simulink model "active_cell_balancing"  (R2021a)
settings: Solver=VariableStepAuto  StartTime=0.0  StopTime=5  RelTol=1e-3
undefined symbols (not defined in the file): Ion, Lithium
libraries: spsIdealSwitchLib x4, spsSeriesRLCBranchLib x4, spsBatteryLib x2, spsDiodeLib x2, spsDCVoltageSourceLib x1, spsGroundLib x1, spsPWMGenerator2LevelLib x1, spspowerguiLib x1
settings Model: Creator=suraj kumar  LastModifiedBy=suraj kumar

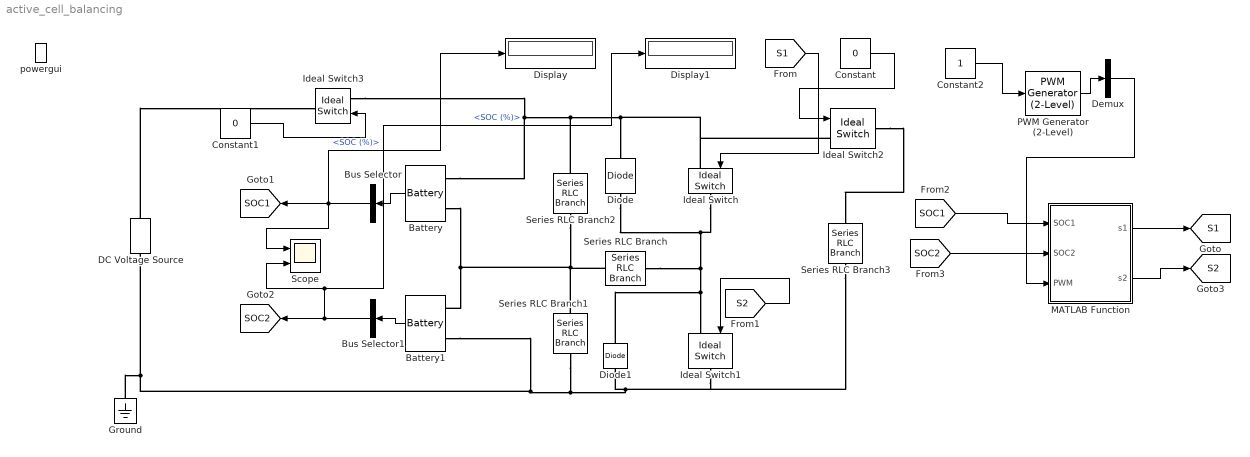
== system active_cell_balancing ==
  Battery : spsBatteryLib/Battery  BatType=Lithium-Ion  ShowTempParam=off  ThermalPreset=no  ShowAgeParam=off  NomV=3.6  NomQ=5.4  SOC=50  Batt_Tr=30  PresetModel=on  MaxQ=5.4  MinV=2.7  FullV=4.1904  Dis_rate=2.3478  R=0.0066667  Normal_OP=4.8835  expZone="[3.8894      0.2653]"  current=[6.5 13 32.5]  Units=Time  Tci=20  NomT=20  T2=-30  MaxQ2=4.8  FullV2=7.1  Normal_OP2=5.655  expZone2="[6.58           1]"  Rca=0.6  ti=2000  Dp=0  Neq0=0  Tsim=1e6  Ta1=25  Qeol=5.4*0.9  Reol=0.013333*1.2  Char_age=[2.3478, 3]  Dis_age=[2.3478, 10]  N1=1500  N2=10500  N3=1000  N4=1400  Ta2=45  N5=950
  Battery1 : spsBatteryLib/Battery  BatType=Lithium-Ion  ShowTempParam=off  ThermalPreset=no  ShowAgeParam=off  NomV=3.7  NomQ=5.4  SOC=60  Batt_Tr=30  PresetModel=on  MaxQ=5.4  MinV=2.775  FullV=4.3068  Dis_rate=2.3478  R=0.0068519  Normal_OP=4.8835  expZone="[3.9974      0.2653]"  current=[6.5 13 32.5]  Units=Time  Tci=20  NomT=20  T2=-30  MaxQ2=4.8  FullV2=7.1  Normal_OP2=5.655  expZone2="[6.58           1]"  Rca=0.6  ti=2000  Dp=0  Neq0=0  Tsim=1e6  Ta1=25  Qeol=5.4*0.9  Reol=0.013333*1.2  Char_age=[2.3478, 3]  Dis_age=[2.3478, 10]  N1=1500  N2=10500  N3=1000  N4=1400  Ta2=45  N5=950
  Bus Selector : BusSelector  OutputSignals=SOC (%)
  Bus Selector1 : BusSelector  OutputSignals=SOC (%)
  Constant : Constant  Value=0
  Constant1 : Constant  Value=0
  Constant2 : Constant
  DC Voltage Source : spsDCVoltageSourceLib/DC Voltage Source  Amplitude=12  Measurements=None
  Demux : Demux  Outputs=1
  Diode : spsDiodeLib/Diode  Ron=0.001  Lon=0  Vf=0.8  IC=0  UseSnubber=0  Rs=500  Cs=250e-9  Measurements=off
  Diode1 : spsDiodeLib/Diode  Ron=0.001  Lon=0  Vf=0.8  IC=0  UseSnubber=0  Rs=500  Cs=250e-9  Measurements=off
  Display : Display
  Display1 : Display
  Ground : spsGroundLib/Ground  LConnTagsString=a
  Ideal Switch{,1..3} (4 alike) : spsIdealSwitchLib/Ideal Switch  Ron=0.001  Lon=0  IC=0  Rs=1e5  Cs=inf  Measurements=off
  MATLAB Function : MATLAB Function  TreatAsAtomicUnit=on
  PWM Generator (2-Level) : spsPWMGenerator2LevelLib/PWM Generator (2-Level)  ModulatorType=Single-phase half-bridge (2 pulses)  ModulatorMode=Unsynchronized  Fc=500  Pc=0  nF=27  MinMax="[ -1  1 ]"  SamplingTechnique=Natural  ModulatingSignals=off  m=0.8  Freq=60  Phase=0  Ts=0  ShowCarrierOutport=off
  Scope : Scope  NumInputPorts=2
  Series RLC Branch : spsSeriesRLCBranchLib/Series RLC Branch  LConnTagsString=__new0  RConnTagsString=__new0  BranchType=L  Resistance=1  Inductance=1e-3  SetiL0=off  InitialCurrent=0  Capacitance=1e-6  Setx0=off  InitialVoltage=0  Measurements=None
  Series RLC Branch1 : spsSeriesRLCBranchLib/Series RLC Branch  LConnTagsString=__new0  RConnTagsString=__new0  BranchType=C  Resistance=1  Inductance=1e-3  SetiL0=off  InitialCurrent=0  Capacitance=1e-6  Setx0=off  InitialVoltage=0  Measurements=None
  Series RLC Branch2 : spsSeriesRLCBranchLib/Series RLC Branch  LConnTagsString=__new0  RConnTagsString=__new0  BranchType=C  Resistance=1  Inductance=1e-3  SetiL0=off  InitialCurrent=0  Capacitance=1e-6  Setx0=off  InitialVoltage=0  Measurements=None
  Series RLC Branch3 : spsSeriesRLCBranchLib/Series RLC Branch  LConnTagsString=__new0  RConnTagsString=__new0  BranchType=R  Resistance=1  Inductance=1e-3  SetiL0=off  InitialCurrent=0  Capacitance=1e-6  Setx0=off  InitialVoltage=0  Measurements=None
  powergui : spspowerguiLib/powergui  Priority=1  SimulationMode=Discrete  SampleTime=50e-5  frequency=60  Iterations=50  frequencyindice=0  Pbase=100e6  ErrMax=1e-4  UnitsV=kV  UnitsW=MW  buscounter=0  FunctionMessages=off  echomessages=off  EnableUseOfTLC=off  CurrentSourceSwitches=off  DisableSnubberDevices=off  DisableRonSwitches=off  DisableVfSwitches=off  DisplayEquations=off  AutomaticDiscreteSolvers=off  SolverType=Tustin/Backward Euler (TBE)  Interpol=off  ExternalGateDelay=off  methode=off  Ts=100  x0status=blocks  SPID=on  SwTol=0  HookPort=off  NonlinearTolerance=1e-4  nMaxIteration=100  ContinueOnMaxIteration=off  RestoreLinks=warning  ResistiveCurrentMeasurement=off  Frange=[0:2:500]  Ylog=off  Xlog=on  ShowGrid=off  save=off  variable=ZData  structure=0  ZoomFFT=off  StartTime=0.0  cycles=1  DisplayStyle=1  fundamental=60  FreqAxis=off  MaxFrequency=1000  frequencyindicesteady=1  RmsSteady=1  display=off
  tag scope: S1=global, S2=global, SOC1=global, SOC2=global
  wires:
  Battery/1 -> Bus Selector/1
  Battery1/1 -> Bus Selector1/1
  Bus Selector/1 -> Scope/1, Display/1, [SOC1]  "<SOC (%)>"
  [S1] -> Ideal Switch/1
  Bus Selector1/1 -> Scope/2, Display1/1, [SOC2]  "<SOC (%)>"
  [S2] -> Ideal Switch1/1
  Constant/1 -> Ideal Switch2/1
  Constant1/1 -> Ideal Switch3/1
  PWM Generator (2-Level)/1 -> Demux/1
  [SOC1] -> MATLAB Function/1(SOC1)
  [SOC2] -> MATLAB Function/2(SOC2)
  Demux/1 -> MATLAB Function/3(PWM)
  MATLAB Function/1(s1) -> [S1]
  MATLAB Function/2(s2) -> [S2]
  Constant2/1 -> PWM Generator (2-Level)/1
  connections:
  Battery/LConn1 -- Ideal Switch3/LConn1 -- Series RLC Branch2/LConn1 -- Ideal Switch2/LConn1 -- Ideal Switch/LConn1 -- Diode/RConn1
  Battery/LConn2 -- Series RLC Branch/RConn1 -- Series RLC Branch1/LConn1 -- Series RLC Branch2/RConn1 -- Battery1/LConn1
  Ideal Switch/RConn1 -- Diode/LConn1 -- Series RLC Branch/LConn1 -- Diode1/RConn1 -- Ideal Switch1/LConn1
  Ideal Switch2/RConn1 -- Series RLC Branch3/LConn1
  DC Voltage Source/RConn1 -- Ideal Switch3/RConn1
  Battery1/LConn2 -- Ground/LConn1 -- DC Voltage Source/LConn1 -- Series RLC Branch1/RConn1 -- Series RLC Branch3/RConn1 -- Ideal Switch1/RConn1 -- Diode1/LConn1

== matlab function active_cell_balancing/MATLAB Function ==
  data: SOC1 input; s1 output; SOC2 input; PWM input; s2 output
function [s1, s2] = fcn(SOC1, SOC2, PWM)
%#codegen
    % This function compares SOC1 and SOC2 and assigns PWM to s1 or s2
    % based on their values.

    if SOC2 < SOC1
        s1 = PWM;
        s2 = 0;
    elseif SOC2 > SOC1
        s2 = PWM;
        s1 = 0;
    else
        s1 = 0;
        s2 = 0;
    end
end
